simulink model "FeedbackLinearizationController"  (R2019b)
settings: Solver=ode23t  StartTime=0.0  StopTime=25  RelTol=1e-3
undefined symbols (not defined in the file): B, b1, b2, C, D, gravity, Kd, Kp, l, q0
settings Model: Creator=ariannagasparri  LastModifiedBy=ariannagasparri

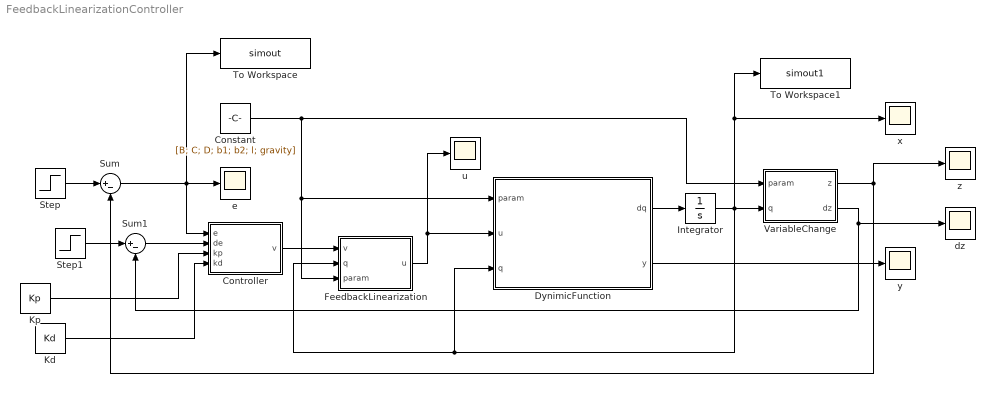
== system FeedbackLinearizationController ==
  Constant : Constant  Value=[B; C; D; b1; b2; l; gravity]
  Controller : MATLAB Function  TreatAsAtomicUnit=on
  DynimicFunction : MATLAB Function  TreatAsAtomicUnit=on
  FeedbackLinearization : MATLAB Function  TreatAsAtomicUnit=on
  Integrator : Integrator  InitialCondition=q0
  Kd : Constant  Value=Kd
  Kp : Constant  Value=Kp
  Step : Step  After=[3,0,0,0]'  SampleTime=0
  Step1 : Step  After=[0,0,0,0]'  SampleTime=0
  Sum : Sum  Inputs=|+-
  Sum1 : Sum  Inputs=|+-
  To Workspace : ToWorkspace  VariableName=simout  SaveFormat=Timeseries  SampleTime=-1
  To Workspace1 : ToWorkspace  VariableName=simout1  SaveFormat=Timeseries  SampleTime=-1
  VariableChange : MATLAB Function  TreatAsAtomicUnit=on
  dz : Scope
  e : Scope
  u : Scope
  x : Scope
  y : Scope
  z : Scope
  wires:
  DynimicFunction/1(dq) -> Integrator/1
  Sum/1 -> To Workspace/1, e/1, Controller/1(e)
  Constant/1 -> VariableChange/1(param), FeedbackLinearization/3(param), DynimicFunction/1(param)
  Step/1 -> Sum/1
  FeedbackLinearization/1(u) -> u/1, DynimicFunction/2(u)
  Integrator/1 -> FeedbackLinearization/2(q), DynimicFunction/3(q), VariableChange/2(q), x/1, To Workspace1/1
  DynimicFunction/2(y) -> y/1
  Controller/1(v) -> FeedbackLinearization/1(v)
  VariableChange/1(z) -> z/1, Sum/2
  Kp/1 -> Controller/3(kp)
  Kd/1 -> Controller/4(kd)
  Step1/1 -> Sum1/1
  Sum1/1 -> Controller/2(de)
  VariableChange/2(dz) -> dz/1, Sum1/2

== matlab function FeedbackLinearizationController/FeedbackLinearization ==
  data: v input; u output; q input; param input
function u = FeedbackLinearization(v, q, param)

B = param(1);
C = param(2);
D = param(3);
b1 = param(4);
b2 = param(5);
l = param(6);
gravity = param(7);

u = (v - Lf2h_fun(B,C,D,b1,b2,gravity,l,q)) / LgLfh_fun(B,C,D,l,q);

end

== matlab function FeedbackLinearizationController/DynimicFunction ==
  data: param input; u input; dq output; q input; y output
function [dq, y] = DynamicFunction(param, u, q)

B = param(1);
C = param(2);
D = param(3);
b1 = param(4);
b2 = param(5);
l = param(6);
gravity = param(7);

dq = f_fun(B,C,D,b1,b2,gravity,l,q) + g_fun(B,C,D,l,q)*u;
y = h_fun(l,q);

end

== matlab function FeedbackLinearizationController/VariableChange ==
  data: param input; q input; z output; dz output
function [z, dz] = VariableChange(param, q)

z = zeros(4,1);
dz = zeros(4,1);

B = param(1);
C = param(2);
D = param(3);
b1 = param(4);
b2 = param(5);
l = param(6);
gravity = param(7);

z(1) = h_fun(l,q);
z(2) = Lfh_fun(l,q);
z(3) = q(1);
z(4) = (-1/(l*cos(q(1))*B))*q(2) + q(4);

dz(1) = z(2);
dz(2) = Lf2h + LgLfh*F;
dz(3) = dq(1);
dz(4) = jacobian(z(4),q)*dq;

end

== matlab function FeedbackLinearizationController/Controller ==
  data: e input; de input; v output; kp input; kd input
function v = Controller(e,de,kp,kd)

v = kp * e + kd * de;

end
